simulink model "etemp"  (R2019a)
settings: Solver=VariableStepAuto  StartTime=0.0  StopTime=10.0  RelTol=1e-3
libraries: nesl_utility x2, fl_lib x1
settings Model: Creator=karth  LastModifiedBy=karth

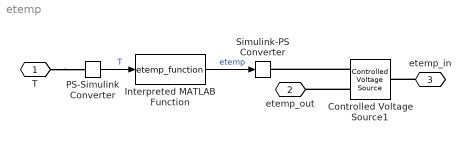
== system etemp ==
  Controlled Voltage Source1 : fl_lib/Electrical/Electrical Sources/Controlled Voltage Source
  Interpreted MATLAB Function : MATLABFcn  MATLABFcn=etemp_function
  PS-Simulink Converter : nesl_utility/PS-Simulink Converter  PhysicalDomain=network_engine_domain  SubClassName=ps_output  LeftPortType=input  RightPortType=output  PseudoPeriodic=off  Frequencies=[]  Unit=1  AffineConversion=off
  Simulink-PS Converter : nesl_utility/Simulink-PS Converter  PhysicalDomain=network_engine_domain  SubClassName=ps_input  LeftPortType=input  RightPortType=output  PseudoPeriodic=off  Frequencies=[]  NoiseDistribution=none  NoiseParameters=[]  Unit=1  AffineConversion=off  FilteringAndDerivatives=provide  SimscapeFilterOrder=1  InputFilterTimeConstant=0.001  UdotUserProvided=0
  T : PMIOPort  Side=Left
  etemp_out : PMIOPort  Port=2  Side=Left
  etemp_in : PMIOPort  Port=3  Side=Left
  wires:
  PS-Simulink Converter/1 -> Interpreted MATLAB Function/1  "T"
  Interpreted MATLAB Function/1 -> Simulink-PS Converter/1  "etemp"
  connections:
  Controlled Voltage Source1/RConn1 -- Simulink-PS Converter/RConn1
  T/RConn1 -- PS-Simulink Converter/LConn1
  Controlled Voltage Source1/RConn2 -- etemp_out/RConn1
  etemp_in/RConn1 -- Controlled Voltage Source1/LConn1
